simulink model "wing_multisine_model"  (R2025b)
settings: Solver=ode4  StartTime=0.0  StopTime=31.9975  FixedStep=0.0025  RelTol=1e-3
InitFcn:
  | wg_ts = multisine_function_generator(); assignin('base','wg_ts',wg_ts);
settings Model: Creator=sek_kim  LastModifiedBy=sek_kim

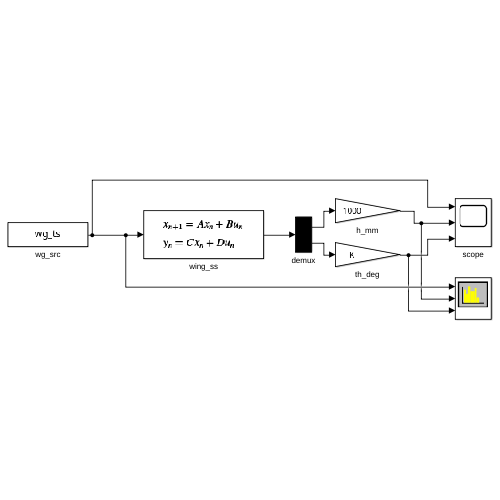
[thumbnail: Simulink's stored preview of the top-level diagram]
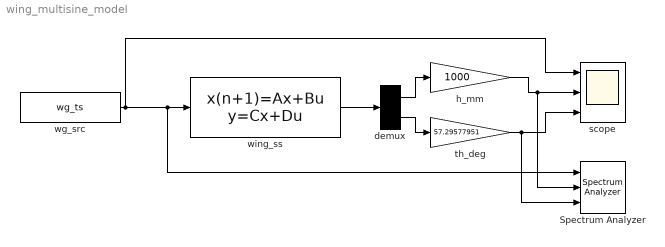
== system wing_multisine_model ==
  Spectrum Analyzer : SpectrumAnalyzer  NumInputPorts=3  WindowPosition=[26.666668,228.000000,342.000000,500.000000,]  ScopeFrameLocation=window  SampleRateSource=Property  SampleRate=400  PlotAsTwoSidedSpectrum=off  FrequencyScale=Log  WindowInvariantSamplesPerUpdate=on  Span=200  CenterFrequency=100  StartFrequency=0  StopFrequency=200  YLimits=[-52.2997 45.3168]
  demux : Demux  Outputs=2
  h_mm : Gain  Gain=1000
  scope : Scope  NumInputPorts=3
      settings: ActiveDisplayYMinimum=-13.82329016200241  ActiveDisplayYMaximum=9.8731573192135151
  th_deg : Gain  Gain=57.29577951
  wg_src : FromWorkspace  VariableName=wg_ts  SampleTime=0.0025
  wing_ss : DiscreteStateSpace  A=[0.99623139189277 -5.25130413244714e-05 0.00247574479951531 1.75616318189352e-07;0.0054909787147955 0.989755465807576 0.000142586384796456 0.00246210203088703;-3.00437689005879 -0.0420347443293541 0.979404510792882 0.000121878264094386;4.30915802158372 -8.15010220195159 0.114911899185891 0.966420769540183]  B=[-1.16878835716856e-05;0.000124240474015212;-0.00931593887474141;0.0986480254171361]  C=[1 0 0 0;0 1 0 0]  D=[0;0]  InitialCondition=[0;0;0;0]  SampleTime=0.0025
  wires:
  wg_src/1 -> Spectrum Analyzer/1, wing_ss/1, scope/1
  wing_ss/1 -> demux/1
  demux/1 -> h_mm/1
  demux/2 -> th_deg/1
  h_mm/1 -> Spectrum Analyzer/2, scope/2
  th_deg/1 -> Spectrum Analyzer/3, scope/3
